simulink model "X_position_CL"  (R2023a)
settings: Solver=FixedStepAuto  StartTime=0.0  StopTime=inf  FixedStep=0.043  RelTol=1e-3
undefined symbols (not defined in the file): Angular, Linear
libraries: robotlib x15
settings Model: Creator=yoav  LastModifiedBy=connectlab
settings SolverCC: InsertRTBMode=Never (minimum delay)
settings OptimizationCC: EnhancedBackFolding=on  PassReuseOutputArgsAs=Individual arguments  ZeroExternalMemoryAtStartup=off  ZeroInternalMemoryAtStartup=off  MaxStackSize=64  OptimizeBlockOrder=speed  DifferentSizesBufferReuse=on  OptimizationCustomize=off  EfficientTunableParamExpr=on
settings DebuggingCC: ParameterTunabilityLossMsg=error
settings HardwareCC: ProdBitPerPointer=32  ProdBitPerSizeT=32  ProdBitPerPtrDiffT=32  ProdLargestAtomicFloat=None  ProdIntDivRoundTo=Undefined  ProdEndianess=Unspecified  ProdWordSize=32  ProdHWDeviceType=Generic->Unspecified (assume 32-bit Generic)
settings SFSimCC: MATLABDynamicMemAlloc=off
settings RTWCC: Description=Embedded Coder  SystemTargetFile=ert.tlc  HardwareBoard=Robot Operating System (ROS)  TLCOptions="-aInlineSetEventsForThisBaseRateFcn=TLC_FALSE -aSuppressMultiTaskScheduler=TLC_FALSE  -aRateBasedStepFcn=0"  TemplateMakefile=ert_default_tmf  Toolchain=Catkin  TargetLang=C++
settings CodeAppCC: ForceParamTrailComments=on  IgnoreCustomStorageClasses=off  OperatorAnnotations=on  SimulinkDataObjDesc=on  SFDataObjDesc=on  InsertBlockDesc=on
settings ERTTargetCC: ExtMode=on  ExtModeMexArgs='192.168.1.155' 0 17725

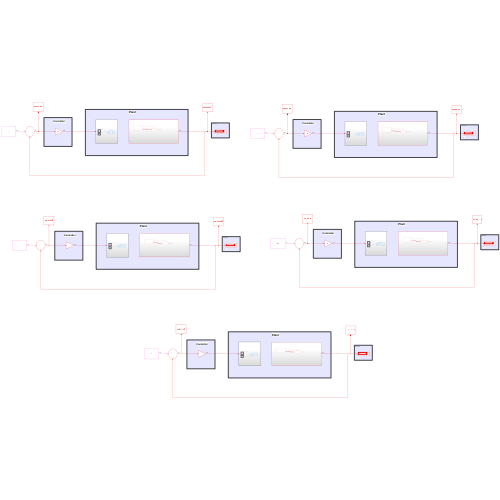
[thumbnail: Simulink's stored preview of the top-level diagram]
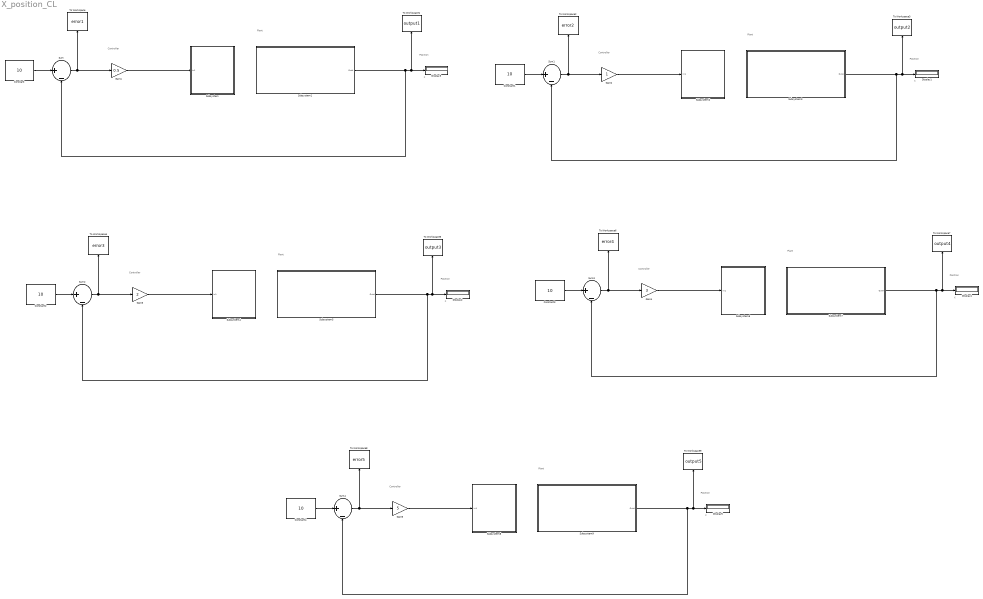
== system X_position_CL ==
  note: Controller
  note: Plant
  note: Position
  note: X
  note: X
  note: Plant
  note: Position
  note: Controller
  note: X
  note: Plant
  note: Position
  note: Controller
  note: Position
  note: Controller
  note: X
  note: Plant
  note: X
  note: Controller
  note: Position
  note: Plant
  Constant{,1..4} (5 alike) : Constant  Value=10
  Display{1..5} (5 alike) : Display
  Gain1 : Gain  Gain=0.5
  Gain2 : Gain
  Gain3 : Gain  Gain=2
  Gain4 : Gain  Gain=3
  Gain5 : Gain  Gain=5
  Subsystem : Subsystem
  Subsystem1 : Subsystem
  Subsystem2 : Subsystem
  Subsystem3 : Subsystem
  Subsystem4 : Subsystem
  Subsystem5 : Subsystem
  Subsystem6 : Subsystem
  Subsystem7 : Subsystem
  Subsystem8 : Subsystem
  Subsystem9 : Subsystem
  Sum{,1..4} (5 alike) : Sum  Inputs=|+-
  To Workspace : ToWorkspace  VariableName=error1  SaveFormat=Timeseries  SampleTime=-1
  To Workspace1 : ToWorkspace  VariableName=output1  SaveFormat=Timeseries  SampleTime=-1
  To Workspace2 : ToWorkspace  VariableName=error2  SaveFormat=Timeseries  SampleTime=-1
  To Workspace3 : ToWorkspace  VariableName=output2  SaveFormat=Timeseries  SampleTime=-1
  To Workspace4 : ToWorkspace  VariableName=error3  SaveFormat=Timeseries  SampleTime=-1
  To Workspace5 : ToWorkspace  VariableName=output3  SaveFormat=Timeseries  SampleTime=-1
  To Workspace6 : ToWorkspace  VariableName=error4  SaveFormat=Timeseries  SampleTime=-1
  To Workspace7 : ToWorkspace  VariableName=output4  SaveFormat=Timeseries  SampleTime=-1
  To Workspace8 : ToWorkspace  VariableName=error5  SaveFormat=Timeseries  SampleTime=-1
  To Workspace9 : ToWorkspace  VariableName=output5  SaveFormat=Timeseries  SampleTime=-1
  wires:
  Subsystem1/1(Out4) -> Sum/2, Display3/1, To Workspace1/1
  Constant/1 -> Sum/1
  Sum/1 -> To Workspace/1, Gain1/1
  Gain1/1 -> Subsystem/1(In1)
  Constant1/1 -> Sum1/1
  Subsystem3/1(Out4) -> Sum1/2, Display1/1, To Workspace3/1
  Gain2/1 -> Subsystem2/1(In1)
  Sum1/1 -> To Workspace2/1, Gain2/1
  Constant2/1 -> Sum2/1
  Subsystem5/1(Out4) -> Sum2/2, Display2/1, To Workspace5/1
  Gain3/1 -> Subsystem4/1(In1)
  Sum2/1 -> To Workspace4/1, Gain3/1
  Gain4/1 -> Subsystem6/1(In1)
  Constant3/1 -> Sum3/1
  Sum3/1 -> To Workspace6/1, Gain4/1
  Subsystem7/1(Out4) -> Sum3/2, Display4/1, To Workspace7/1
  Gain5/1 -> Subsystem8/1(In1)
  Constant4/1 -> Sum4/1
  Subsystem9/1(Out4) -> Sum4/2, Display5/1, To Workspace9/1
  Sum4/1 -> To Workspace8/1, Gain5/1

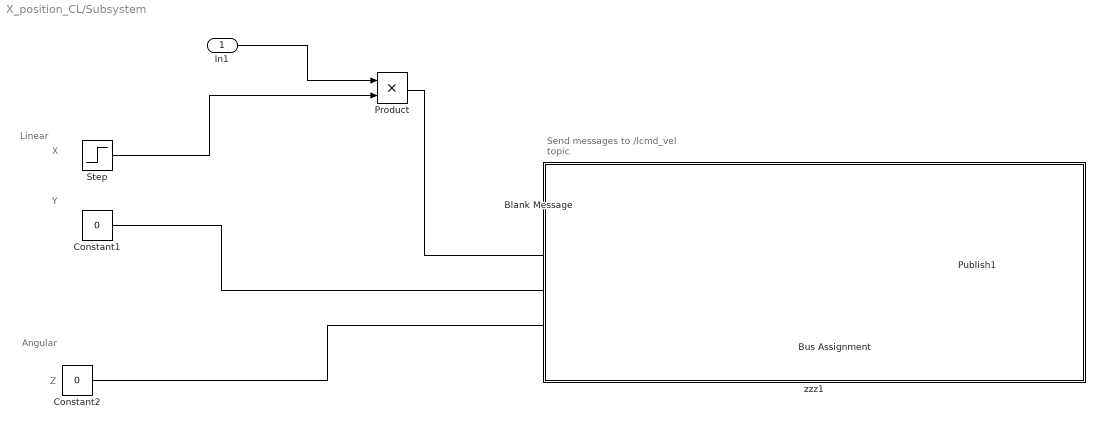
== system X_position_CL/Subsystem ==
  note: Send messages to /lcmd_vel topic
  note: Y
  note: X
  note: Linear
  note: Angular
  note: Z
  In1 : Inport
  Blank Message : robotlib/Blank Message  messageClass=Message  entityType=geometry_msgs/Twist  messageType=geometry_msgs/Twist  SampleTime=inf  legacyBusStruct=off
  Bus Assignment : BusAssignment  AssignedSignals=Linear.X,Linear.Y,Angular.Z
  Constant1 : Constant  Value=0
  Constant2 : Constant  Value=0
  Product : Product
  Publish1 : robotlib/Publish  topicSource=Specify your own  topic=/robot1/cmd_vel  messageType=geometry_msgs/Twist  legacyBusStruct=off  messageQueueLength=105
  Step : Step  Time=0  SampleTime=0
  zzz1 : Subsystem  TreatAsAtomicUnit=on
      settings: OpenFcn=% no-op
      mask Display: disp('')
  wires:
  Blank Message/1 -> Bus Assignment/1
  Bus Assignment/1 -> Publish1/1
  Constant2/1 -> Bus Assignment/4
  Constant1/1 -> Bus Assignment/3
  In1/1 -> Product/1
  Step/1 -> Product/2
  Product/1 -> Bus Assignment/2

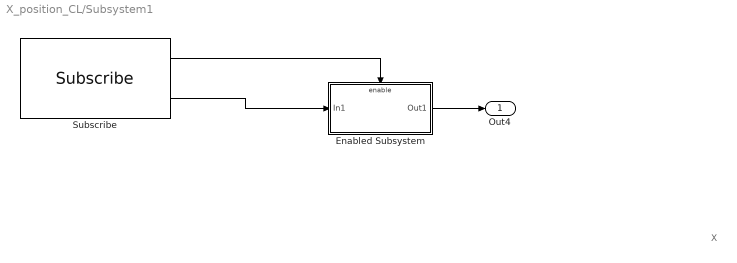
== system X_position_CL/Subsystem1 ==
  note: X
  Enabled Subsystem : Subsystem  TreatAsAtomicUnit=on
  Subscribe : robotlib/Subscribe  topicSource=Select from ROS network  topic=/robot1/odom  messageType=nav_msgs/Odometry  SampleTime=-1  legacyBusStruct=off  messageQueueLength=1
      settings: LibrarySourceBlock=roslib/ROS/Subscribe
  Out4 : Outport
  wires:
  Subscribe/2 -> Enabled Subsystem/1(In1)
  Subscribe/1 -> Enabled Subsystem/Enable
  Enabled Subsystem/1(Out1) -> Out4/1

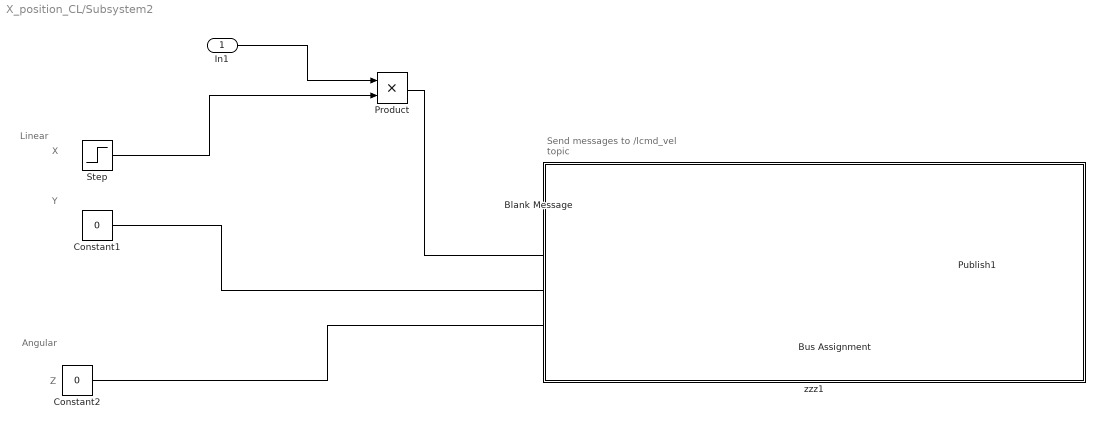
== system X_position_CL/Subsystem2 ==
  note: Send messages to /lcmd_vel topic
  note: Y
  note: X
  note: Linear
  note: Angular
  note: Z
  In1 : Inport
  Blank Message : robotlib/Blank Message  messageClass=Message  entityType=geometry_msgs/Twist  messageType=geometry_msgs/Twist  SampleTime=inf  legacyBusStruct=off
  Bus Assignment : BusAssignment  AssignedSignals=Linear.X,Linear.Y,Angular.Z
  Constant1 : Constant  Value=0
  Constant2 : Constant  Value=0
  Product : Product
  Publish1 : robotlib/Publish  topicSource=Specify your own  topic=/robot2/cmd_vel  messageType=geometry_msgs/Twist  legacyBusStruct=off  messageQueueLength=105
  Step : Step  Time=0  SampleTime=0
  zzz1 : Subsystem  TreatAsAtomicUnit=on
      settings: OpenFcn=% no-op
      mask Display: disp('')
  wires:
  Blank Message/1 -> Bus Assignment/1
  Bus Assignment/1 -> Publish1/1
  Constant2/1 -> Bus Assignment/4
  Constant1/1 -> Bus Assignment/3
  In1/1 -> Product/1
  Step/1 -> Product/2
  Product/1 -> Bus Assignment/2

== system X_position_CL/Subsystem3 ==
  note: X
  Enabled Subsystem : Subsystem  TreatAsAtomicUnit=on
  Subscribe : robotlib/Subscribe  topicSource=Select from ROS network  topic=/robot2/odom  messageType=nav_msgs/Odometry  SampleTime=-1  legacyBusStruct=off  messageQueueLength=1
      settings: LibrarySourceBlock=roslib/ROS/Subscribe
  Out4 : Outport
  wires:
  Subscribe/2 -> Enabled Subsystem/1(In1)
  Subscribe/1 -> Enabled Subsystem/Enable
  Enabled Subsystem/1(Out1) -> Out4/1

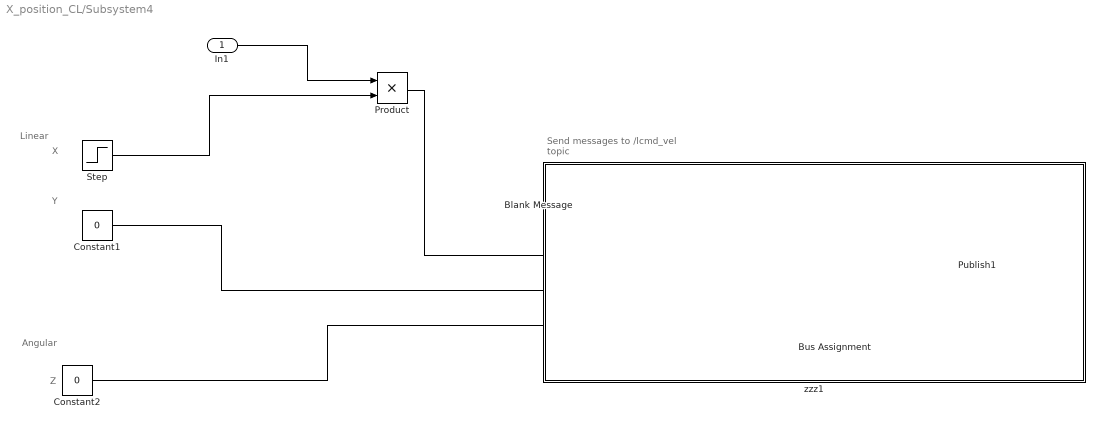
== system X_position_CL/Subsystem4 ==
  note: Send messages to /lcmd_vel topic
  note: Y
  note: X
  note: Linear
  note: Angular
  note: Z
  In1 : Inport
  Blank Message : robotlib/Blank Message  messageClass=Message  entityType=geometry_msgs/Twist  messageType=geometry_msgs/Twist  SampleTime=inf  legacyBusStruct=off
  Bus Assignment : BusAssignment  AssignedSignals=Linear.X,Linear.Y,Angular.Z
  Constant1 : Constant  Value=0
  Constant2 : Constant  Value=0
  Product : Product
  Publish1 : robotlib/Publish  topicSource=Specify your own  topic=/robot3/cmd_vel  messageType=geometry_msgs/Twist  legacyBusStruct=off  messageQueueLength=105
  Step : Step  Time=0  SampleTime=0
  zzz1 : Subsystem  TreatAsAtomicUnit=on
      settings: OpenFcn=% no-op
      mask Display: disp('')
  wires:
  Blank Message/1 -> Bus Assignment/1
  Bus Assignment/1 -> Publish1/1
  Constant2/1 -> Bus Assignment/4
  Constant1/1 -> Bus Assignment/3
  In1/1 -> Product/1
  Step/1 -> Product/2
  Product/1 -> Bus Assignment/2

== system X_position_CL/Subsystem5 ==
  note: X
  Enabled Subsystem : Subsystem  TreatAsAtomicUnit=on
  Subscribe : robotlib/Subscribe  topicSource=Select from ROS network  topic=/robot3/odom  messageType=nav_msgs/Odometry  SampleTime=-1  legacyBusStruct=off  messageQueueLength=1
      settings: LibrarySourceBlock=roslib/ROS/Subscribe
  Out4 : Outport
  wires:
  Subscribe/2 -> Enabled Subsystem/1(In1)
  Subscribe/1 -> Enabled Subsystem/Enable
  Enabled Subsystem/1(Out1) -> Out4/1

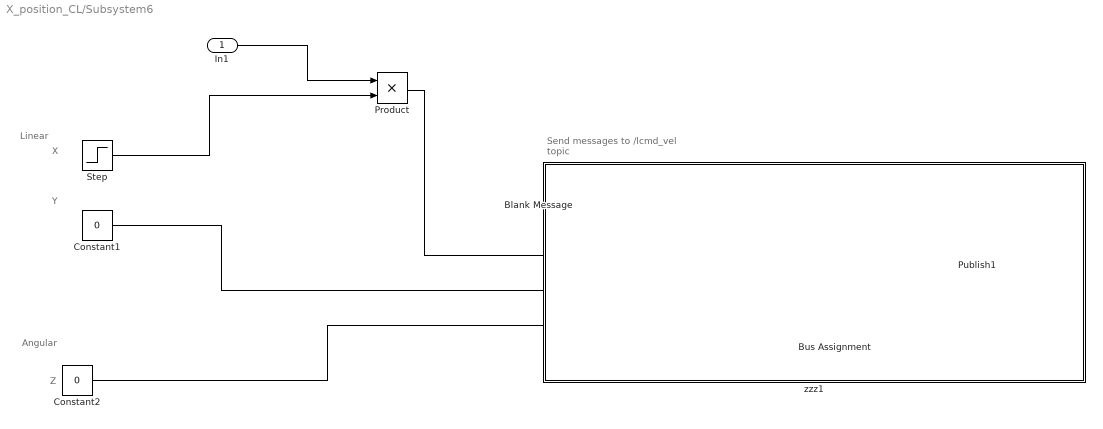
== system X_position_CL/Subsystem6 ==
  note: Send messages to /lcmd_vel topic
  note: Y
  note: X
  note: Linear
  note: Angular
  note: Z
  In1 : Inport
  Blank Message : robotlib/Blank Message  messageClass=Message  entityType=geometry_msgs/Twist  messageType=geometry_msgs/Twist  SampleTime=inf  legacyBusStruct=off
  Bus Assignment : BusAssignment  AssignedSignals=Linear.X,Linear.Y,Angular.Z
  Constant1 : Constant  Value=0
  Constant2 : Constant  Value=0
  Product : Product
  Publish1 : robotlib/Publish  topicSource=Specify your own  topic=/robot4/cmd_vel  messageType=geometry_msgs/Twist  legacyBusStruct=off  messageQueueLength=105
  Step : Step  Time=0  SampleTime=0
  zzz1 : Subsystem  TreatAsAtomicUnit=on
      settings: OpenFcn=% no-op
      mask Display: disp('')
  wires:
  Blank Message/1 -> Bus Assignment/1
  Bus Assignment/1 -> Publish1/1
  Constant2/1 -> Bus Assignment/4
  Constant1/1 -> Bus Assignment/3
  In1/1 -> Product/1
  Step/1 -> Product/2
  Product/1 -> Bus Assignment/2

== system X_position_CL/Subsystem7 ==
  note: X
  Enabled Subsystem : Subsystem  TreatAsAtomicUnit=on
  Subscribe : robotlib/Subscribe  topicSource=Select from ROS network  topic=/robot4/odom  messageType=nav_msgs/Odometry  SampleTime=-1  legacyBusStruct=off  messageQueueLength=1
      settings: LibrarySourceBlock=roslib/ROS/Subscribe
  Out4 : Outport
  wires:
  Subscribe/2 -> Enabled Subsystem/1(In1)
  Subscribe/1 -> Enabled Subsystem/Enable
  Enabled Subsystem/1(Out1) -> Out4/1

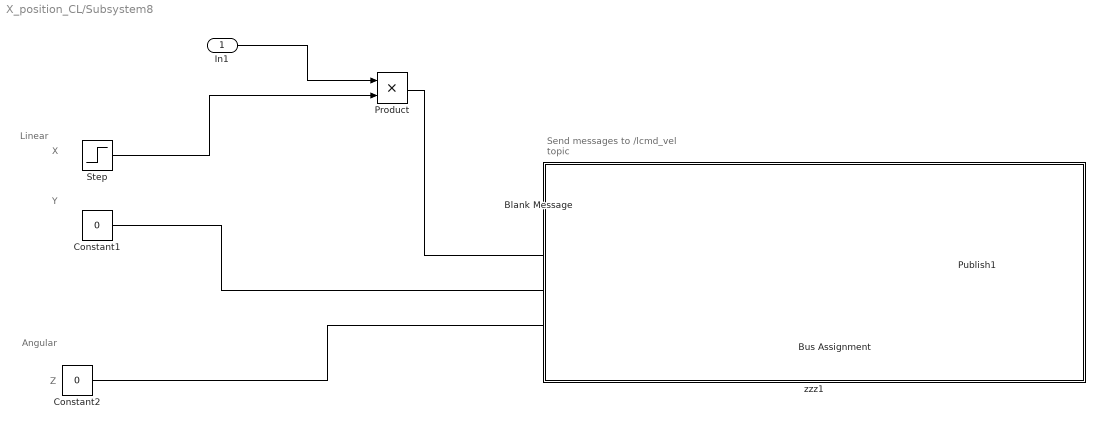
== system X_position_CL/Subsystem8 ==
  note: Send messages to /lcmd_vel topic
  note: Y
  note: X
  note: Linear
  note: Angular
  note: Z
  In1 : Inport
  Blank Message : robotlib/Blank Message  messageClass=Message  entityType=geometry_msgs/Twist  messageType=geometry_msgs/Twist  SampleTime=inf  legacyBusStruct=off
  Bus Assignment : BusAssignment  AssignedSignals=Linear.X,Linear.Y,Angular.Z
  Constant1 : Constant  Value=0
  Constant2 : Constant  Value=0
  Product : Product
  Publish1 : robotlib/Publish  topicSource=Specify your own  topic=/robot5/cmd_vel  messageType=geometry_msgs/Twist  legacyBusStruct=off  messageQueueLength=105
  Step : Step  Time=0  SampleTime=0
  zzz1 : Subsystem  TreatAsAtomicUnit=on
      settings: OpenFcn=% no-op
      mask Display: disp('')
  wires:
  Blank Message/1 -> Bus Assignment/1
  Bus Assignment/1 -> Publish1/1
  Constant2/1 -> Bus Assignment/4
  Constant1/1 -> Bus Assignment/3
  In1/1 -> Product/1
  Step/1 -> Product/2
  Product/1 -> Bus Assignment/2

== system X_position_CL/Subsystem9 ==
  note: X
  Enabled Subsystem : Subsystem  TreatAsAtomicUnit=on
  Subscribe : robotlib/Subscribe  topicSource=Select from ROS network  topic=/robot5/odom  messageType=nav_msgs/Odometry  SampleTime=-1  legacyBusStruct=off  messageQueueLength=1
      settings: LibrarySourceBlock=roslib/ROS/Subscribe
  Out4 : Outport
  wires:
  Subscribe/2 -> Enabled Subsystem/1(In1)
  Subscribe/1 -> Enabled Subsystem/Enable
  Enabled Subsystem/1(Out1) -> Out4/1

== system X_position_CL/Subsystem/zzz1 ==

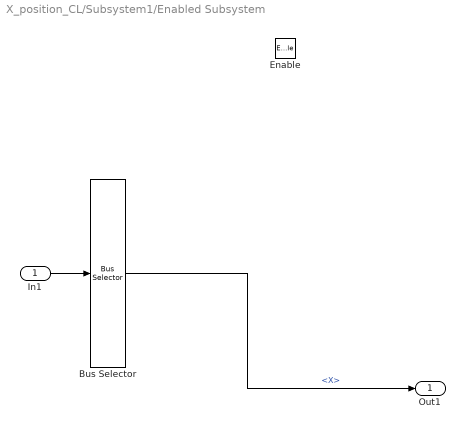
== system X_position_CL/Subsystem1/Enabled Subsystem ==
  In1 : Inport
  Enable : EnablePort
  Bus Selector : BusSelector  OutputSignals=Pose.Pose.Position.X
  Out1 : Outport
  wires:
  In1/1 -> Bus Selector/1
  Bus Selector/1 -> Out1/1  "<X>"

== system X_position_CL/Subsystem2/zzz1 ==

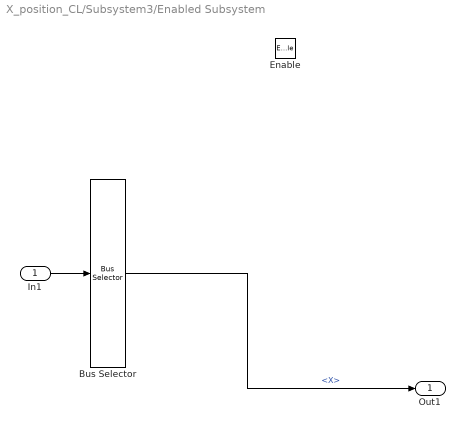
== system X_position_CL/Subsystem3/Enabled Subsystem ==
  In1 : Inport
  Enable : EnablePort
  Bus Selector : BusSelector  OutputSignals=Pose.Pose.Position.X
  Out1 : Outport
  wires:
  In1/1 -> Bus Selector/1
  Bus Selector/1 -> Out1/1  "<X>"

== system X_position_CL/Subsystem4/zzz1 ==

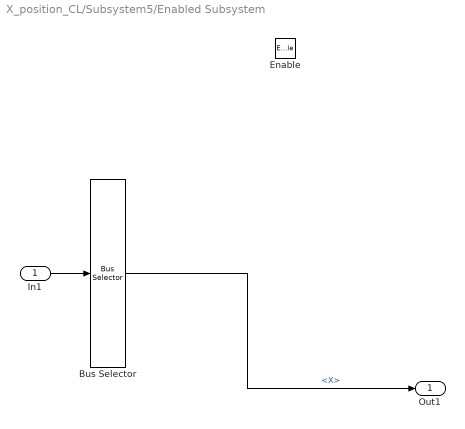
== system X_position_CL/Subsystem5/Enabled Subsystem ==
  In1 : Inport
  Enable : EnablePort
  Bus Selector : BusSelector  OutputSignals=Pose.Pose.Position.X
  Out1 : Outport
  wires:
  In1/1 -> Bus Selector/1
  Bus Selector/1 -> Out1/1  "<X>"

== system X_position_CL/Subsystem6/zzz1 ==

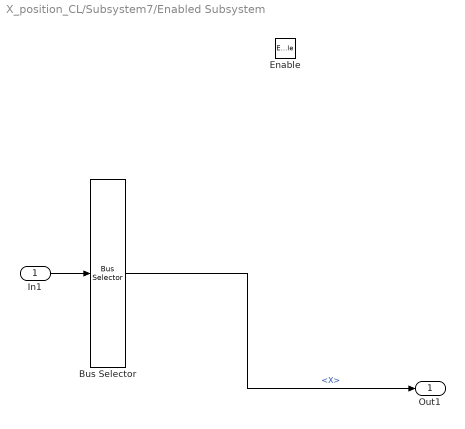
== system X_position_CL/Subsystem7/Enabled Subsystem ==
  In1 : Inport
  Enable : EnablePort
  Bus Selector : BusSelector  OutputSignals=Pose.Pose.Position.X
  Out1 : Outport
  wires:
  In1/1 -> Bus Selector/1
  Bus Selector/1 -> Out1/1  "<X>"

== system X_position_CL/Subsystem8/zzz1 ==

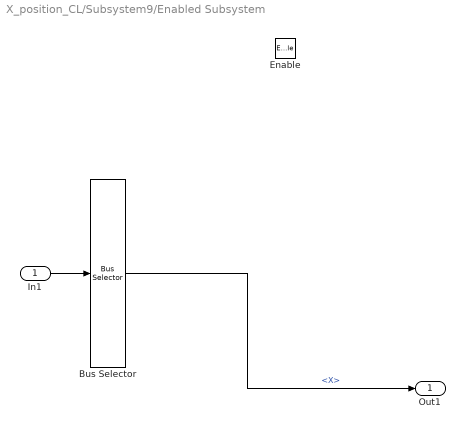
== system X_position_CL/Subsystem9/Enabled Subsystem ==
  In1 : Inport
  Enable : EnablePort
  Bus Selector : BusSelector  OutputSignals=Pose.Pose.Position.X
  Out1 : Outport
  wires:
  In1/1 -> Bus Selector/1
  Bus Selector/1 -> Out1/1  "<X>"
